simulink model "modelisation_paroi_multi_4"  (R2019b)
settings: Solver=VariableStepAuto  StartTime=0.0  StopTime=48*3600  RelTol=1e-3
undefined symbols (not defined in the file): kse, ksi, lam_1, lam_2, lam_3, S, T_ext, T_int
libraries: fl_lib x28, nesl_utility x4
settings Model: Creator=Ivan  LastModifiedBy=Ivan

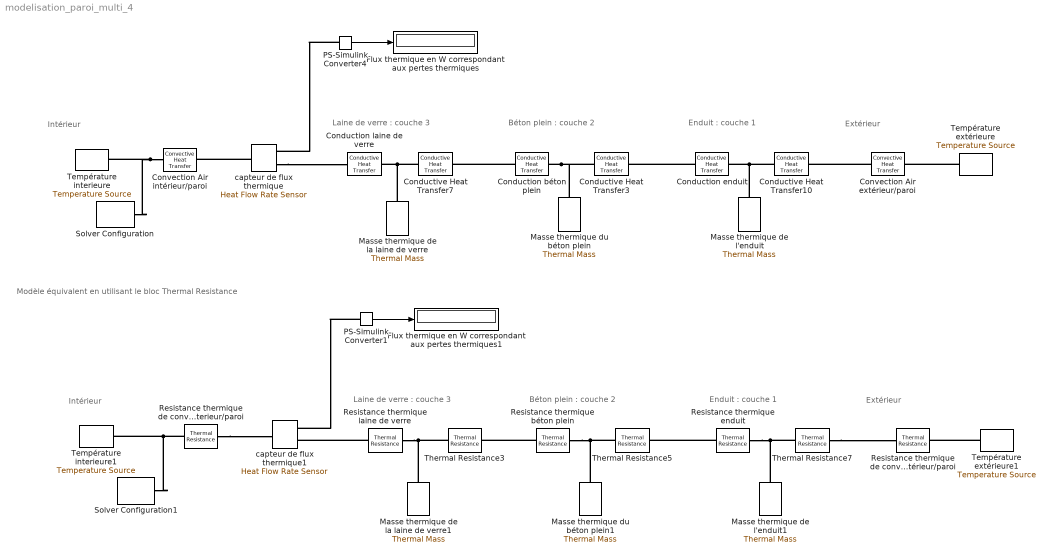
== system modelisation_paroi_multi_4 ==
  note: Modèle équivalent en utilisant le bloc Thermal Resistance
  note: Extérieur
  note: Intérieur
  note: Béton plein : couche 2
  note: Laine de verre : couche 3
  note: Enduit : couche 1
  note: Extérieur
  note: Intérieur
  note: Béton plein : couche 2
  note: Laine de verre : couche 3
  note: Enduit : couche 1
  Conduction laine de verre : fl_lib/Thermal/Thermal Elements/Conductive Heat Transfer  area=S m^2  thickness=e3/2 cm  th_cond=lam_3 W/(m*K)  T_specify=off  T_priority=None  T=0 K  T_nominal_specify=off  T_nominal_unit=K  T_nominal_value=1  Q_specify=off  Q_priority=None  Q=0 W  Q_nominal_specify=off  Q_nominal_unit=W  Q_nominal_value=1
      settings: SourceProductName=Simscape
  Conduction béton plein : fl_lib/Thermal/Thermal Elements/Conductive Heat Transfer  area=S m^2  thickness=e2/2 cm  th_cond=lam_2 W/(m*K)  T_specify=off  T_priority=None  T=0 K  T_nominal_specify=off  T_nominal_unit=K  T_nominal_value=1  Q_specify=off  Q_priority=None  Q=0 W  Q_nominal_specify=off  Q_nominal_unit=W  Q_nominal_value=1
      settings: SourceProductName=Simscape
  Conduction enduit : fl_lib/Thermal/Thermal Elements/Conductive Heat Transfer  area=S m^2  thickness=e1/2 cm  th_cond=lam_1 W/(m*K)  T_specify=off  T_priority=None  T=0 K  T_nominal_specify=off  T_nominal_unit=K  T_nominal_value=1  Q_specify=off  Q_priority=None  Q=0 W  Q_nominal_specify=off  Q_nominal_unit=W  Q_nominal_value=1
      settings: SourceProductName=Simscape
  Conductive Heat Transfer10 : fl_lib/Thermal/Thermal Elements/Conductive Heat Transfer  area=S m^2  thickness=e1/2 cm  th_cond=lam_1 W/(m*K)  T_specify=off  T_priority=None  T=0 K  T_nominal_specify=off  T_nominal_unit=K  T_nominal_value=1  Q_specify=off  Q_priority=None  Q=0 W  Q_nominal_specify=off  Q_nominal_unit=W  Q_nominal_value=1
      settings: SourceProductName=Simscape
  Conductive Heat Transfer3 : fl_lib/Thermal/Thermal Elements/Conductive Heat Transfer  area=S m^2  thickness=e2/2 cm  th_cond=lam_2 W/(m*K)  T_specify=off  T_priority=None  T=0 K  T_nominal_specify=off  T_nominal_unit=K  T_nominal_value=1  Q_specify=off  Q_priority=None  Q=0 W  Q_nominal_specify=off  Q_nominal_unit=W  Q_nominal_value=1
      settings: SourceProductName=Simscape
  Conductive Heat Transfer7 : fl_lib/Thermal/Thermal Elements/Conductive Heat Transfer  area=S m^2  thickness=e3/2 cm  th_cond=lam_3 W/(m*K)  T_specify=off  T_priority=None  T=0 K  T_nominal_specify=off  T_nominal_unit=K  T_nominal_value=1  Q_specify=off  Q_priority=None  Q=0 W  Q_nominal_specify=off  Q_nominal_unit=W  Q_nominal_value=1
      settings: SourceProductName=Simscape
  Convection Air extérieur/paroi : fl_lib/Thermal/Thermal Elements/Convective Heat Transfer  area=S m^2  heat_tr_coeff=kse W/(m^2 * K)  T_specify=off  T_priority=None  T=0 K  T_nominal_specify=off  T_nominal_unit=K  T_nominal_value=1  Q_specify=off  Q_priority=None  Q=0 W  Q_nominal_specify=off  Q_nominal_unit=W  Q_nominal_value=1
  Convection Air intérieur/paroi : fl_lib/Thermal/Thermal Elements/Convective Heat Transfer  area=S m^2  heat_tr_coeff=ksi W/(m^2 * K)  T_specify=off  T_priority=None  T=0 K  T_nominal_specify=off  T_nominal_unit=K  T_nominal_value=1  Q_specify=off  Q_priority=None  Q=0 W  Q_nominal_specify=off  Q_nominal_unit=W  Q_nominal_value=1
  Flux thermique en W correspondant aux pertes thermiques : Display
  Flux thermique en W correspondant aux pertes thermiques1 : Display
  Masse thermique de la laine de verre : fl_lib/Thermal/Thermal Elements/Thermal Mass  mass=m3 kg  sp_heat=c3 J/kg/K  T_specify=on  T_priority=High  T=T_int degC  T_nominal_specify=off  T_nominal_unit=K  T_nominal_value=1  Q_specify=off  Q_priority=None  Q=0 W  Q_nominal_specify=off  Q_nominal_unit=W  Q_nominal_value=1
  Masse thermique de la laine de verre1 : fl_lib/Thermal/Thermal Elements/Thermal Mass  mass=m3 kg  sp_heat=c3 J/kg/K  T_specify=on  T_priority=High  T=T_int degC  T_nominal_specify=off  T_nominal_unit=K  T_nominal_value=1  Q_specify=off  Q_priority=None  Q=0 W  Q_nominal_specify=off  Q_nominal_unit=W  Q_nominal_value=1
  Masse thermique de l'enduit : fl_lib/Thermal/Thermal Elements/Thermal Mass  mass=m1 kg  sp_heat=c1 J/kg/K  T_specify=on  T_priority=High  T=T_ext degC  T_nominal_specify=off  T_nominal_unit=K  T_nominal_value=1  Q_specify=off  Q_priority=None  Q=0 W  Q_nominal_specify=off  Q_nominal_unit=W  Q_nominal_value=1
  Masse thermique de l'enduit1 : fl_lib/Thermal/Thermal Elements/Thermal Mass  mass=m1 kg  sp_heat=c1 J/kg/K  T_specify=on  T_priority=High  T=T_ext degC  T_nominal_specify=off  T_nominal_unit=K  T_nominal_value=1  Q_specify=off  Q_priority=None  Q=0 W  Q_nominal_specify=off  Q_nominal_unit=W  Q_nominal_value=1
  Masse thermique du béton plein : fl_lib/Thermal/Thermal Elements/Thermal Mass  mass=m2 kg  sp_heat=c2 J/kg/K  T_specify=on  T_priority=High  T=(T_int+T_ext)/2 degC  T_nominal_specify=off  T_nominal_unit=K  T_nominal_value=1  Q_specify=off  Q_priority=None  Q=0 W  Q_nominal_specify=off  Q_nominal_unit=W  Q_nominal_value=1
  Masse thermique du béton plein1 : fl_lib/Thermal/Thermal Elements/Thermal Mass  mass=m2 kg  sp_heat=c2 J/kg/K  T_specify=on  T_priority=High  T=(T_int+T_ext)/2 degC  T_nominal_specify=off  T_nominal_unit=K  T_nominal_value=1  Q_specify=off  Q_priority=None  Q=0 W  Q_nominal_specify=off  Q_nominal_unit=W  Q_nominal_value=1
  PS-Simulink Converter1 : nesl_utility/PS-Simulink Converter  PhysicalDomain=network_engine_domain  SubClassName=ps_output  LeftPortType=input  RightPortType=output  PseudoPeriodic=off  Frequencies=[]  Unit=W  AffineConversion=off
  PS-Simulink Converter4 : nesl_utility/PS-Simulink Converter  PhysicalDomain=network_engine_domain  SubClassName=ps_output  LeftPortType=input  RightPortType=output  PseudoPeriodic=off  Frequencies=[]  Unit=W  AffineConversion=off
  Resistance thermique de convection AIr interieur/paroi : fl_lib/Thermal/Thermal Elements/Thermal Resistance  resistance=1/(ksi*S) K/W  T_specify=off  T_priority=None  T=0 K  T_nominal_specify=off  T_nominal_unit=K  T_nominal_value=1  Q_specify=off  Q_priority=None  Q=0 W  Q_nominal_specify=off  Q_nominal_unit=W  Q_nominal_value=1
      settings: SourceProductName=Simscape  SourceProductBaseCode=SS
  Resistance thermique laine de verre : fl_lib/Thermal/Thermal Elements/Thermal Resistance  resistance=((e3/2)*1e-2)/(lam_3*S) K/W  T_specify=off  T_priority=None  T=0 K  T_nominal_specify=off  T_nominal_unit=K  T_nominal_value=1  Q_specify=off  Q_priority=None  Q=0 W  Q_nominal_specify=off  Q_nominal_unit=W  Q_nominal_value=1
      settings: SourceProductName=Simscape  SourceProductBaseCode=SS
  Resistance thermique enduit : fl_lib/Thermal/Thermal Elements/Thermal Resistance  resistance=((e1/2)*1e-2)/(lam_1*S) K/W  T_specify=off  T_priority=None  T=0 K  T_nominal_specify=off  T_nominal_unit=K  T_nominal_value=1  Q_specify=off  Q_priority=None  Q=0 W  Q_nominal_specify=off  Q_nominal_unit=W  Q_nominal_value=1
      settings: SourceProductName=Simscape  SourceProductBaseCode=SS
  Resistance thermique béton plein : fl_lib/Thermal/Thermal Elements/Thermal Resistance  resistance=((e2/2)*1e-2)/(lam_2*S) K/W  T_specify=off  T_priority=None  T=0 K  T_nominal_specify=off  T_nominal_unit=K  T_nominal_value=1  Q_specify=off  Q_priority=None  Q=0 W  Q_nominal_specify=off  Q_nominal_unit=W  Q_nominal_value=1
      settings: SourceProductName=Simscape  SourceProductBaseCode=SS
  Resistance thermique de convection AIr extérieur/paroi : fl_lib/Thermal/Thermal Elements/Thermal Resistance  resistance=1/(kse*S) K/W  T_specify=off  T_priority=None  T=0 K  T_nominal_specify=off  T_nominal_unit=K  T_nominal_value=1  Q_specify=off  Q_priority=None  Q=0 W  Q_nominal_specify=off  Q_nominal_unit=W  Q_nominal_value=1
      settings: SourceProductName=Simscape  SourceProductBaseCode=SS
  Solver Configuration : nesl_utility/Solver Configuration  PhysicalDomain=network_engine_domain  SubClassName=solver  LeftPortType=input  RightPortType=generic  Tones=[]  Harmonics=[]  SimulateNoise=off  Profile=off  UseLocalSampling=off  EnableSwitchedLinearOptims=on  FrequencyDomain=off  UseCCode=off  RelTol=0.001  AbsTol=1e-06  MinStep=1e-09  ToWorkspace=off  RevertToSquareIcSolve=off  NumHomotopyIterations=100  PhasorMode=off  PhasorModeNumHarmonics=1  DoDC=off  ResidualTolerance=1e-09  UseLocalSolver=off  LocalSolverChoice=NE_BACKWARD_EULER_ADVANCER  LocalSolverSampleTime=0.001  DoFixedCost=off  MaxNonlinIter=3  MaxModeIter=2  LinearAlgebra=auto  EquationFormulation=NE_TIME_EF  DelaysMemoryBudget=1024  AutomaticFiltering=on  FilteringTimeConstant=0.001  PartitionStorageMethod=AS_NEEDED  PartitionMemoryBudget=1024  PartitionMethod=ROBUST
  Solver Configuration1 : nesl_utility/Solver Configuration  PhysicalDomain=network_engine_domain  SubClassName=solver  LeftPortType=input  RightPortType=generic  Tones=[]  Harmonics=[]  SimulateNoise=off  Profile=off  UseLocalSampling=off  EnableSwitchedLinearOptims=on  FrequencyDomain=off  UseCCode=off  RelTol=0.001  AbsTol=1e-06  MinStep=1e-09  ToWorkspace=off  RevertToSquareIcSolve=off  NumHomotopyIterations=100  PhasorMode=off  PhasorModeNumHarmonics=1  DoDC=off  ResidualTolerance=1e-09  UseLocalSolver=off  LocalSolverChoice=NE_BACKWARD_EULER_ADVANCER  LocalSolverSampleTime=0.001  DoFixedCost=off  MaxNonlinIter=3  MaxModeIter=2  LinearAlgebra=auto  EquationFormulation=NE_TIME_EF  DelaysMemoryBudget=1024  AutomaticFiltering=on  FilteringTimeConstant=0.001  PartitionStorageMethod=AS_NEEDED  PartitionMemoryBudget=1024  PartitionMethod=ROBUST
  Température extérieure : fl_lib/Thermal/Thermal Sources/Temperature Source  temperature=T_ext degC
      settings: SourceProductName=Simscape
  Température extérieure1 : fl_lib/Thermal/Thermal Sources/Temperature Source  temperature=T_ext degC
      settings: SourceProductName=Simscape
  Température interieure : fl_lib/Thermal/Thermal Sources/Temperature Source  temperature=T_int degC
      settings: SourceProductName=Simscape
  Température interieure1 : fl_lib/Thermal/Thermal Sources/Temperature Source  temperature=T_int degC
      settings: SourceProductName=Simscape
  Thermal Resistance3 : fl_lib/Thermal/Thermal Elements/Thermal Resistance  resistance=((e3/2)*1e-2)/(lam_3*S) K/W  T_specify=off  T_priority=None  T=0 K  T_nominal_specify=off  T_nominal_unit=K  T_nominal_value=1  Q_specify=off  Q_priority=None  Q=0 W  Q_nominal_specify=off  Q_nominal_unit=W  Q_nominal_value=1
      settings: SourceProductName=Simscape  SourceProductBaseCode=SS
  Thermal Resistance5 : fl_lib/Thermal/Thermal Elements/Thermal Resistance  resistance=((e2/2)*1e-2)/(lam_2*S) K/W  T_specify=off  T_priority=None  T=0 K  T_nominal_specify=off  T_nominal_unit=K  T_nominal_value=1  Q_specify=off  Q_priority=None  Q=0 W  Q_nominal_specify=off  Q_nominal_unit=W  Q_nominal_value=1
      settings: SourceProductName=Simscape  SourceProductBaseCode=SS
  Thermal Resistance7 : fl_lib/Thermal/Thermal Elements/Thermal Resistance  resistance=((e1/2)*1e-2)/(lam_1*S) K/W  T_specify=off  T_priority=None  T=0 K  T_nominal_specify=off  T_nominal_unit=K  T_nominal_value=1  Q_specify=off  Q_priority=None  Q=0 W  Q_nominal_specify=off  Q_nominal_unit=W  Q_nominal_value=1
      settings: SourceProductName=Simscape  SourceProductBaseCode=SS
  capteur de flux thermique : fl_lib/Thermal/Thermal Sensors/Heat Flow Rate Sensor
      settings: SourceProductName=Simscape  SourceProductBaseCode=SS
  capteur de flux thermique1 : fl_lib/Thermal/Thermal Sensors/Heat Flow Rate Sensor
      settings: SourceProductName=Simscape  SourceProductBaseCode=SS
  wires:
  PS-Simulink Converter4/1 -> Flux thermique en W correspondant aux pertes thermiques/1
  PS-Simulink Converter1/1 -> Flux thermique en W correspondant aux pertes thermiques1/1
  connections:
  Conduction béton plein/RConn1 -- Masse thermique du béton plein/LConn1 -- Conductive Heat Transfer3/LConn1
  Convection Air intérieur/paroi/LConn1 -- Solver Configuration/RConn1 -- Température interieure/LConn1
  Température extérieure/LConn1 -- Convection Air extérieur/paroi/RConn1
  Masse thermique de la laine de verre/LConn1 -- Conductive Heat Transfer7/LConn1 -- Conduction laine de verre/RConn1
  Conduction béton plein/LConn1 -- Conductive Heat Transfer7/RConn1
  Masse thermique de l'enduit/LConn1 -- Conductive Heat Transfer10/LConn1 -- Conduction enduit/RConn1
  Conduction enduit/LConn1 -- Conductive Heat Transfer3/RConn1
  Convection Air extérieur/paroi/LConn1 -- Conductive Heat Transfer10/RConn1
  capteur de flux thermique/LConn1 -- Convection Air intérieur/paroi/RConn1
  capteur de flux thermique/RConn2 -- Conduction laine de verre/LConn1
  PS-Simulink Converter4/LConn1 -- capteur de flux thermique/RConn1
  Thermal Resistance5/LConn1 -- Masse thermique du béton plein1/LConn1 -- Resistance thermique béton plein/RConn1
  Solver Configuration1/RConn1 -- Température interieure1/LConn1 -- Resistance thermique de convection AIr interieur/paroi/LConn1
  Thermal Resistance3/LConn1 -- Masse thermique de la laine de verre1/LConn1 -- Resistance thermique laine de verre/RConn1
  Thermal Resistance7/LConn1 -- Masse thermique de l'enduit1/LConn1 -- Resistance thermique enduit/RConn1
  PS-Simulink Converter1/LConn1 -- capteur de flux thermique1/RConn1
  Resistance thermique de convection AIr interieur/paroi/RConn1 -- capteur de flux thermique1/LConn1
  Thermal Resistance7/RConn1 -- Resistance thermique de convection AIr extérieur/paroi/LConn1
  Resistance thermique béton plein/LConn1 -- Thermal Resistance3/RConn1
  Resistance thermique laine de verre/LConn1 -- capteur de flux thermique1/RConn2
  Température extérieure1/LConn1 -- Resistance thermique de convection AIr extérieur/paroi/RConn1
  Resistance thermique enduit/LConn1 -- Thermal Resistance5/RConn1
